simulink model "Stateflowques2"  (R2024b)
settings: Solver=VariableStepAuto  StartTime=0.0  StopTime=10.0  RelTol=1e-3

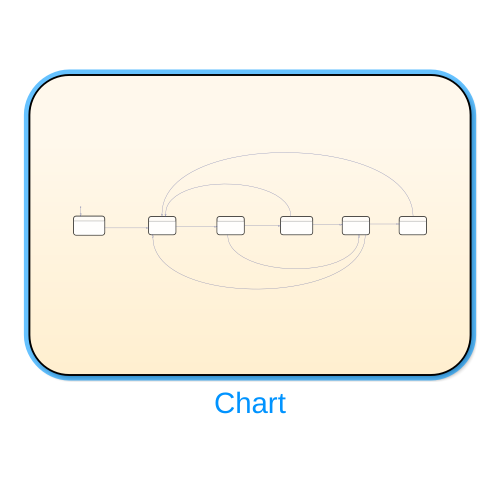
[thumbnail: Simulink's stored preview of the top-level diagram]
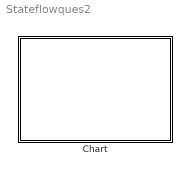
== system Stateflowques2 ==
  Chart : Stateflow chart  TreatAsAtomicUnit=on

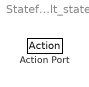
== system Stateflowques2/Chart/Fault_state ==
  Action Port : ActionPort
      settings: CopyFcn=Stateflow.SLINSF.SimulinkMan.removeBlockPreDeleteFcn  PreDeleteFcn=Stateflow.SLINSF.SimulinkMan.unsafePredeleteFcn

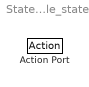
== system Stateflowques2/Chart/Idle_state ==
  Action Port : ActionPort
      settings: CopyFcn=Stateflow.SLINSF.SimulinkMan.removeBlockPreDeleteFcn  PreDeleteFcn=Stateflow.SLINSF.SimulinkMan.unsafePredeleteFcn

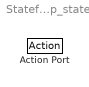
== system Stateflowques2/Chart/Sleep_state ==
  Action Port : ActionPort
      settings: CopyFcn=Stateflow.SLINSF.SimulinkMan.removeBlockPreDeleteFcn  PreDeleteFcn=Stateflow.SLINSF.SimulinkMan.unsafePredeleteFcn

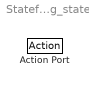
== system Stateflowques2/Chart/charging_state ==
  Action Port : ActionPort
      settings: CopyFcn=Stateflow.SLINSF.SimulinkMan.removeBlockPreDeleteFcn  PreDeleteFcn=Stateflow.SLINSF.SimulinkMan.unsafePredeleteFcn

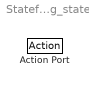
== system Stateflowques2/Chart/discharging_state ==
  Action Port : ActionPort
      settings: CopyFcn=Stateflow.SLINSF.SimulinkMan.removeBlockPreDeleteFcn  PreDeleteFcn=Stateflow.SLINSF.SimulinkMan.unsafePredeleteFcn

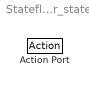
== system Stateflowques2/Chart/monitor_state ==
  Action Port : ActionPort
      settings: CopyFcn=Stateflow.SLINSF.SimulinkMan.removeBlockPreDeleteFcn  PreDeleteFcn=Stateflow.SLINSF.SimulinkMan.unsafePredeleteFcn

== stateflow chart Stateflowques2/Chart ==
  state Idle_state
  state monitor_state
  state charging_state
  state discharging_state
  state Fault_state
  state Sleep_state
  Sleep_state -> monitor_state : [systemActive]
  discharging_state -> monitor_state [order 2] : [chargingComplete && voltageSafe && currentSafe]
  (default) -> Idle_state
  Fault_state -> Sleep_state [order 1] : [~systemActive
      | ]
  discharging_state -> Fault_state [order 1] : [(after(0.5, sec) && (~voltageSafe || ~currentSafe)) || (after(1, sec) && (temperature > 60))
      | ]
  charging_state -> discharging_state [order 1] : [chargerDisconnected && batteryInUse && voltageSafe && currentSafe && temperatureSafe]
  monitor_state -> charging_state : [chargerConnected && voltageSafe && currentSafe && temperatureSafe]
  Idle_state -> monitor_state : [systemON || chargerConnected]
  Fault_state -> monitor_state [order 2] : [after(0.5, sec) && voltageSafe && currentSafe && after(1, sec) && temperature <= 60]
  charging_state -> Fault_state [order 2] : [~voltageSafe || ~currentSafe || ~temperatureSafe]
  data: sf_internal_action_state_placeholder_data local double size=1 =0; sf_internal_action_state_placeholder_data local double size=1 =0; sf_internal_action_state_placeholder_data local double size=1 =0; sf_internal_action_state_placeholder_data local double size=1 =0; sf_internal_action_state_placeholder_data local double size=1 =0; sf_internal_action_state_placeholder_data local double size=1 =0
